simulink model "Super11"  (Simulink 5.0)
settings: Solver=ode45  StartTime=0.0  StopTime=10.0  RelTol=1e-3
settings Model: Creator=scaife  LastModifiedBy=scaife  ExtModeAutoUpdateStatusClock=off

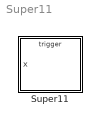
== system Super11 ==
  Super11 : Stateflow chart

== stateflow chart Super11 ==
  state A
  state B
    state B1
    state B2
      state B2a
      (default) -> B2a
      B2a -> (junction 9) : E
    B1 -> B2 : E
    (default) -> B1
    (junction 9) -> B1 : [x<>0]
  (default) -> A
  A -> (junction 8) : E
  (junction 9) -> A : [x==0]
  (junction 8) -> B : [x==0]
  (junction 8) -> B2a : [x<>0]
  data: x input int32
  events: E input EITHER_EDGE_EVENT
